simulink model "back_emf"  (R2022b)
settings: Solver=VariableStepAuto  StartTime=0.0  StopTime=0.05  FixedStep=0.0000001  RelTol=1e-3
libraries: spsDCVoltageSourceLib x1, spsGroundLib x1, spsPermanentMagnetSynchronousMachineLib x1, spsSVPWMGenerator2LevelLib x1, spsThreePhaseParallelRLCBranchLib x1, spsUniversalBridgeLib x1, spsVoltageMeasurementLib x1, spsdq0toAlphaBetaZeroLib x1, spspowerguiLib x1
settings Model: Creator=ZJX  LastModifiedBy=ZJX

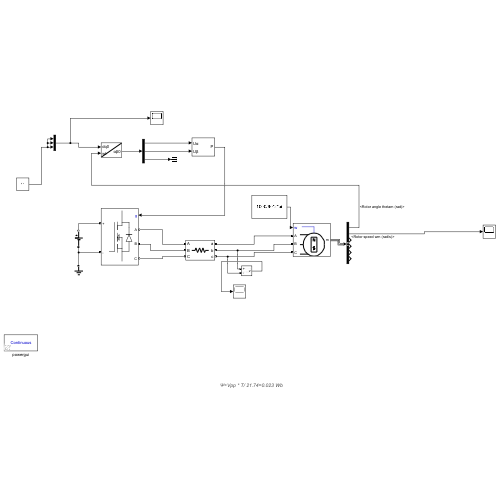
[thumbnail: Simulink's stored preview of the top-level diagram]
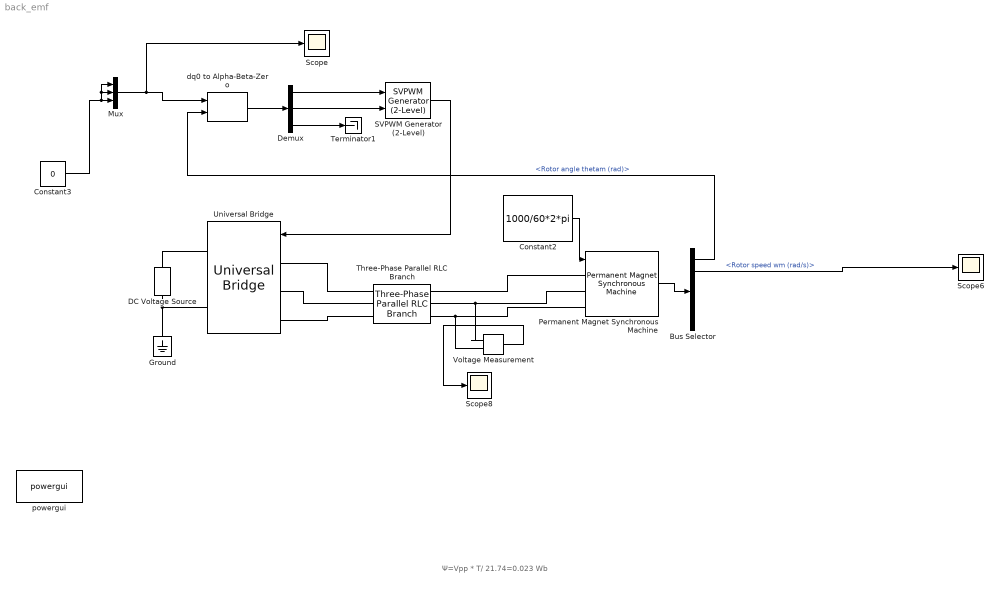
== system back_emf ==
  note: Ψ=Vpp * T/ 21.74=0.023 Wb
  Bus Selector : BusSelector  OutputSignals=Rotor angle thetam (rad),Rotor speed wm (rad/s),Stator current is_a (A),Stator current is_b (A),Stator current is_c (A),Electromagnetic torque Te (N*m)
  Constant2 : Constant  Value=1000/60*2*pi
  Constant3 : Constant  Value=0
  DC Voltage Source : spsDCVoltageSourceLib/DC Voltage Source  Amplitude=24  Measurements=None
  Demux : Demux  Outputs=3
  Ground : spsGroundLib/Ground  LConnTagsString=a
  Mux : Mux  Inputs=3
  Permanent Magnet Synchronous Machine : spsPermanentMagnetSynchronousMachineLib/Permanent Magnet Synchronous Machine  NbPhases=3  FluxDistribution=Sinusoidal  RotorType=Round  MechanicalLoad=Speed w  PresetModel=No  ShowDetailedParameters=on  MeasurementBus=off  Resistance=0.1  Inductance=8.5e-3  dqInductances=[8.5e-3,8.5e-3]  La=0.00017  MachineConstant=Flux linkage established by magnets (V.s)  Flux=0.05  VoltageCst=9.069  TorqueCst=0.075  Flat=120  Mechanical=[0.00027 0.0004924 1 0]  PolePairs=1  InitialConditions=[0,0, 0,0]  InitialConditions5ph=[0 0 0 0 0 0]  RefAngle=90 degrees behind phase A axis (modified Park)  IterativeDiscreteModel=Trapezoidal non iterative  TsBlock=-1  TsPowergui=0
  SVPWM Generator (2-Level) : spsSVPWMGenerator2LevelLib/SVPWM Generator (2-Level)  InputType=alpha-beta components  SwitchingPattern=Pattern #1  Fc=20000  ParUref=[0.8 -30 50]  Ts=0
  Scope : Scope
  Scope6 : Scope
  Scope8 : Scope
  Terminator1 : Terminator
  Three-Phase Parallel RLC Branch : spsThreePhaseParallelRLCBranchLib/Three-Phase Parallel RLC Branch  LConnTagsString=A|B|C  RConnTagsString=A|B|C  BranchType=R  Resistance=10000  Inductance=1e-3  Capacitance=1e-6  Measurements=None
  Universal Bridge : spsUniversalBridgeLib/Universal Bridge  Arms=3  SnubberResistance=1e5  SnubberCapacitance=inf  Device=MOSFET / Diodes  Ron=10000000  Lon=0  ForwardVoltages="[  0  0  ]"  ForwardVoltage=0  GTOparameters=[ 10e-6 , 20e-6 ]  IGBTparameters=[ 1e-6 , 2e-6 ]  Measurements=None  Measurements_2=None  converterType=Rectifier
  Voltage Measurement : spsVoltageMeasurementLib/Voltage Measurement  PhasorSimulation=off  OutputType=Complex  PSBequivalent=0
  dq0 to Alpha-Beta-Zero : spsdq0toAlphaBetaZeroLib/dq0 to Alpha-Beta-Zero  Alignment=90 degrees behind phase A axis
  powergui : spspowerguiLib/powergui  Priority=1  SimulationMode=Continuous  SampleTime=0.000025  frequency=60  Iterations=50  frequencyindice=0  Pbase=100e6  ErrMax=1e-4  UnitsV=kV  UnitsW=MW  buscounter=0  FunctionMessages=off  echomessages=off  EnableUseOfTLC=off  CurrentSourceSwitches=off  DisableSnubberDevices=off  DisableRonSwitches=off  DisableVfSwitches=off  DisplayEquations=off  AutomaticDiscreteSolvers=off  SolverType=Tustin/Backward Euler (TBE)  Interpol=off  ExternalGateDelay=off  methode=off  Ts=100  x0status=blocks  SPID=on  SwTol=0  HookPort=off  NonlinearTolerance=1e-4  nMaxIteration=100  ContinueOnMaxIteration=off  RestoreLinks=warning  ResistiveCurrentMeasurement=off  Frange=[0:2:500]  Ylog=off  Xlog=on  ShowGrid=off  save=off  variable=ZData  structure=0  ZoomFFT=off  StartTime=0.0  cycles=1  DisplayStyle=1  fundamental=60  FreqAxis=off  MaxFrequency=1000  frequencyindicesteady=1  RmsSteady=1  display=off
  wires:
  Demux/3 -> Terminator1/1
  Bus Selector/2 -> Scope6/1  "<Rotor speed wm (rad/s)>"
  SVPWM Generator (2-Level)/1 -> Universal Bridge/1
  Mux/1 -> Scope/1, dq0 to Alpha-Beta-Zero/1
  Permanent Magnet Synchronous Machine/1 -> Bus Selector/1
  Demux/2 -> SVPWM Generator (2-Level)/2
  dq0 to Alpha-Beta-Zero/1 -> Demux/1
  Bus Selector/1 -> dq0 to Alpha-Beta-Zero/2  "<Rotor angle thetam (rad)>"
  Demux/1 -> SVPWM Generator (2-Level)/1
  Constant2/1 -> Permanent Magnet Synchronous Machine/1
  Voltage Measurement/1 -> Scope8/1
  Constant3/1 -> Mux/1, Mux/2, Mux/3
  connections:
  Ground/LConn1 -- Universal Bridge/RConn2 -- DC Voltage Source/LConn1
  DC Voltage Source/RConn1 -- Universal Bridge/RConn1
  Three-Phase Parallel RLC Branch/RConn1 -- Permanent Magnet Synchronous Machine/LConn1
  Three-Phase Parallel RLC Branch/LConn1 -- Universal Bridge/LConn1
  Three-Phase Parallel RLC Branch/LConn2 -- Universal Bridge/LConn2
  Three-Phase Parallel RLC Branch/RConn2 -- Voltage Measurement/LConn1 -- Permanent Magnet Synchronous Machine/LConn2
  Three-Phase Parallel RLC Branch/LConn3 -- Universal Bridge/LConn3
  Three-Phase Parallel RLC Branch/RConn3 -- Voltage Measurement/LConn2 -- Permanent Magnet Synchronous Machine/LConn3
